simulink model "pemfc_lumpekf2_prerun_2"  (R2021b)
settings: Solver=ode3  StartTime=0.0  StopTime=10  FixedStep=0.001  MaxStep=dt  RelTol=1e-6
values from neighbouring files (symbols this model uses):
  Optparameter = [kp,kd,ki,b,m1,m2,delta]    [OptGain.m]
  P0 = diag([10,10,10000,10000,10000])    [input_sine.m]    (also in input_step.m)
  x0 = [0.21;0.21;1;1;1]    [OptGain.m]    (also in input_sine.m = [xch_O2c;xch_O2c;J_ss;J_ss;J_ss]; input_step.m = [xch_O2c;xch_O2c;J_ss;J_ss;J_ss])
  xhat0 = [0;0;0;0;0]    [input_sine.m]    (also in input_step.m)
settings Model: Creator=kvijayar  LastModifiedBy=AlirezaBeigi
settings SolverCC: AlgebraicLoopSolver=TrustRegion
settings DataIOCC: InitialState=AA
settings DebuggingCC: SFMachineParentedDataDiag=warning

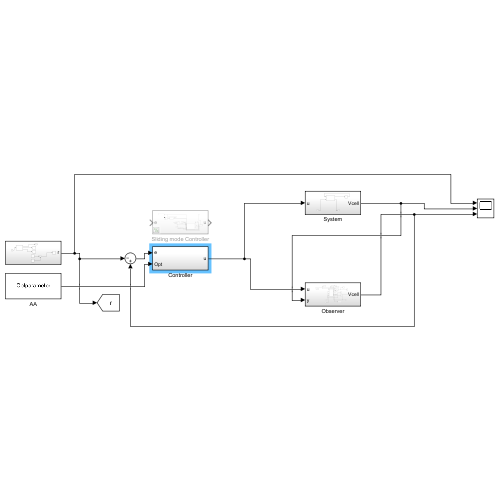
[thumbnail: Simulink's stored preview of the top-level diagram]
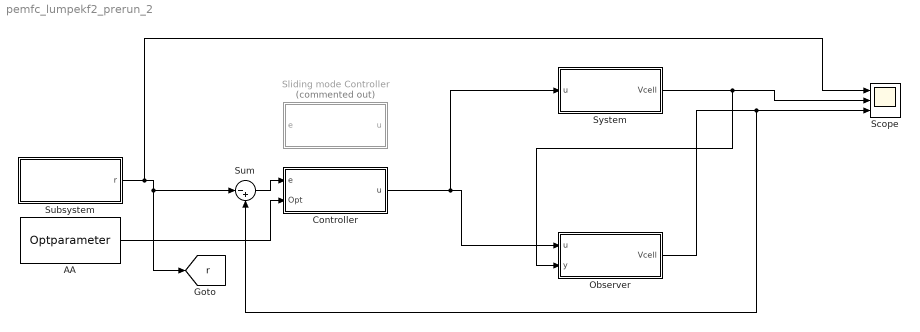
== system pemfc_lumpekf2_prerun_2 ==
  AA : Constant  Value=Optparameter  SampleTime=-1
  Controller : Subsystem  Tag=Controller  Description=Controller
  Observer : Subsystem
  Scope : Scope  NumInputPorts=3
  Sliding mode Controller : Subsystem  Commented=on
  Subsystem : Subsystem
  Sum : Sum  Inputs=|-+
  System : Subsystem
  tag scope: r=global
  wires:
  System/1(Vcell) -> Scope/2, Observer/2(y)
  Observer/1(Vcell) -> Scope/3, Sum/2
  Subsystem/1(r) -> Scope/1, Sum/1, [r]
  Sum/1 -> Controller/1(e)
  Controller/1(u) -> System/1(u), Observer/1(u)
  AA/1 -> Controller/2(Opt)

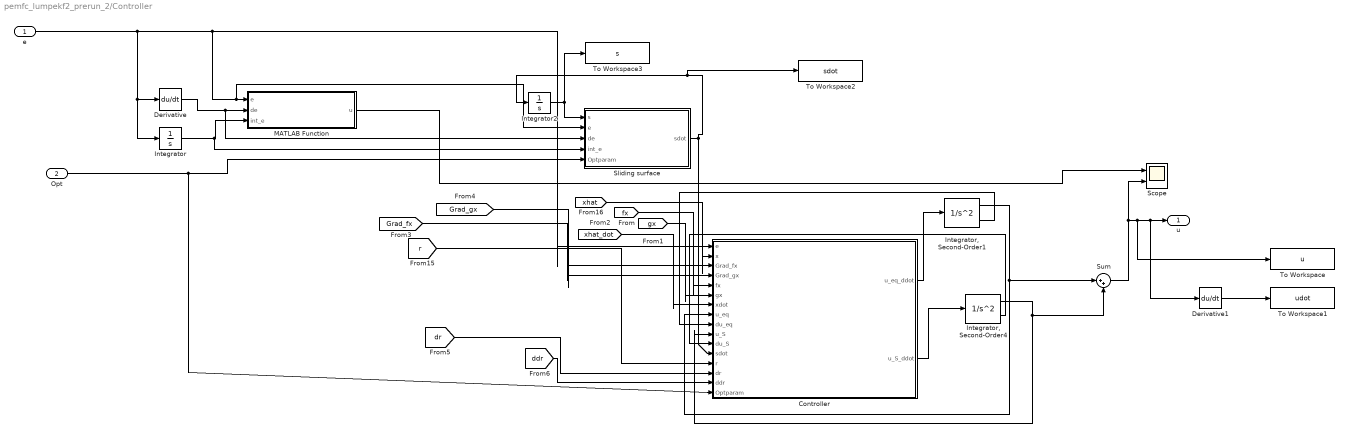
== system pemfc_lumpekf2_prerun_2/Controller ==
  e : Inport
  Opt : Inport  Port=2
  Controller : MATLAB Function  TreatAsAtomicUnit=on
  Derivative : Derivative  CoefficientInTFapproximation=0
  Derivative1 : Derivative  CoefficientInTFapproximation=0
  Integrator : Integrator
  "Integrator, Second-Order1" : SecondOrderIntegrator  ICX=8
  "Integrator, Second-Order4" : SecondOrderIntegrator
  Integrator2 : Integrator
  MATLAB Function : MATLAB Function  TreatAsAtomicUnit=on
  Scope : Scope  NumInputPorts=2
  Sliding surface : MATLAB Function  TreatAsAtomicUnit=on
  Sum : Sum  Inputs=|++
  To Workspace : ToWorkspace  VariableName=u  SaveFormat=Timeseries  SampleTime=-1
  To Workspace1 : ToWorkspace  VariableName=udot  SaveFormat=Timeseries  SampleTime=-1
  To Workspace2 : ToWorkspace  VariableName=sdot  SaveFormat=Timeseries  SampleTime=-1
  To Workspace3 : ToWorkspace  VariableName=s  SaveFormat=Timeseries  SampleTime=-1
  u : Outport
  wires:
  e/1 -> Controller/1(e), Sliding surface/2(e), MATLAB Function/1(e), Integrator/1, Derivative/1
  Derivative/1 -> Sliding surface/3(de), MATLAB Function/2(de)
  Integrator/1 -> Sliding surface/4(int_e), MATLAB Function/3(int_e)
  Integrator2/1 -> To Workspace3/1, Sliding surface/1(s)
  [r] -> Controller/13(r)
  [xhat] -> Controller/2(x)
  Controller/1(u_eq_ddot) -> "Integrator, Second-Order1"/1
  Controller/2(u_S_ddot) -> "Integrator, Second-Order4"/1
  "Integrator, Second-Order4"/1 -> Sum/2, Controller/10(u_S)
  "Integrator, Second-Order4"/2 -> Controller/11(du_S)
  [fx] -> Controller/5(fx)
  [gx] -> Controller/6(gx)
  [xhat_dot] -> Controller/7(xdot)
  [Grad_gx] -> Controller/4(Grad_gx)
  [Grad_fx] -> Controller/3(Grad_fx)
  "Integrator, Second-Order1"/1 -> Sum/1, Controller/8(u_eq)
  "Integrator, Second-Order1"/2 -> Controller/9(du_eq)
  [ddr] -> Controller/15(ddr)
  [dr] -> Controller/14(dr)
  MATLAB Function/1(u) -> Scope/1
  Sum/1 -> To Workspace/1, Derivative1/1, u/1, Scope/2
  Derivative1/1 -> To Workspace1/1
  Sliding surface/1(sdot) -> To Workspace2/1, Integrator2/1, Controller/12(sdot)
  Opt/1 -> Controller/16(Optparam), Sliding surface/5(Optparam)

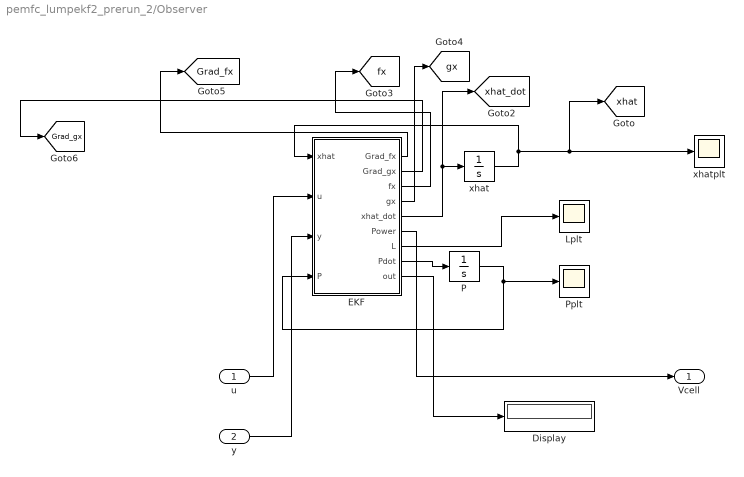
== system pemfc_lumpekf2_prerun_2/Observer ==
  u : Inport
  y : Inport  Port=2
  Display : Display
  EKF : MATLAB Function  TreatAsAtomicUnit=on
  Lplt : Scope
  P : Integrator  InitialCondition=P0
  Pplt : Scope
  xhat : Integrator  InitialCondition=xhat0
  xhatplt : Scope
  Vcell : Outport
  tag scope: Grad_fx=global, Grad_gx=global, fx=global, gx=global, xhat=global, xhat_dot=global
  wires:
  EKF/8(Pdot) -> P/1
  P/1 -> Pplt/1, EKF/4(P)
  xhat/1 -> [xhat], xhatplt/1, EKF/1(xhat)
  EKF/5(xhat_dot) -> [xhat_dot], xhat/1
  EKF/7(L) -> Lplt/1
  EKF/6(Power) -> Vcell/1
  u/1 -> EKF/2(u)
  y/1 -> EKF/3(y)
  EKF/3(fx) -> [fx]
  EKF/4(gx) -> [gx]
  EKF/1(Grad_fx) -> [Grad_fx]
  EKF/2(Grad_gx) -> [Grad_gx]
  EKF/9(out) -> Display/1

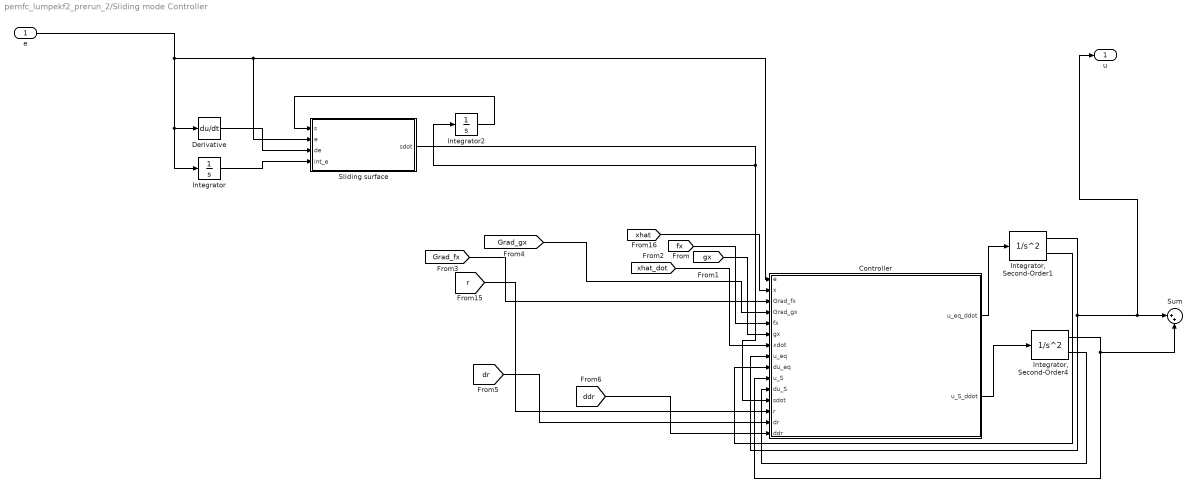
== system pemfc_lumpekf2_prerun_2/Sliding mode Controller ==
  e : Inport
  Controller : MATLAB Function  TreatAsAtomicUnit=on
  Derivative : Derivative  CoefficientInTFapproximation=0
  Integrator : Integrator
  "Integrator, Second-Order1" : SecondOrderIntegrator  AbsoluteToleranceX=0.01
  "Integrator, Second-Order4" : SecondOrderIntegrator
  Integrator2 : Integrator
  Sliding surface : MATLAB Function  TreatAsAtomicUnit=on
  Sum : Sum  Inputs=|++
  u : Outport
  wires:
  Derivative/1 -> Sliding surface/3(de)
  "Integrator, Second-Order1"/1 -> u/1, Sum/1, Controller/8(u_eq)
  [ddr] -> Controller/15(ddr)
  "Integrator, Second-Order1"/2 -> Controller/9(du_eq)
  [Grad_fx] -> Controller/3(Grad_fx)
  [dr] -> Controller/14(dr)
  [gx] -> Controller/6(gx)
  Controller/1(u_eq_ddot) -> "Integrator, Second-Order1"/1
  Controller/2(u_S_ddot) -> "Integrator, Second-Order4"/1
  [fx] -> Controller/5(fx)
  [Grad_gx] -> Controller/4(Grad_gx)
  [xhat] -> Controller/2(x)
  "Integrator, Second-Order4"/1 -> Sum/2, Controller/10(u_S)
  "Integrator, Second-Order4"/2 -> Controller/11(du_S)
  Integrator2/1 -> Sliding surface/1(s)
  [xhat_dot] -> Controller/7(xdot)
  Integrator/1 -> Sliding surface/4(int_e)
  [r] -> Controller/13(r)
  Sliding surface/1(sdot) -> Controller/12(sdot), Integrator2/1
  e/1 -> Controller/1(e), Sliding surface/2(e), Integrator/1, Derivative/1

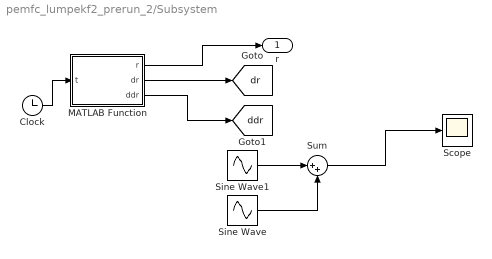
== system pemfc_lumpekf2_prerun_2/Subsystem ==
  Clock : Clock
  MATLAB Function : MATLAB Function  TreatAsAtomicUnit=on
  Scope : Scope
  Sine Wave : Sin  Amplitude=3  Bias=4  Frequency=4  SampleTime=0
  Sine Wave1 : Sin  Amplitude=5  Bias=2  Frequency=2  SampleTime=0
  Sum : Sum  Inputs=|++
  r : Outport
  tag scope: ddr=global, dr=global
  wires:
  Sine Wave1/1 -> Sum/1
  Sine Wave/1 -> Sum/2
  Sum/1 -> Scope/1
  Clock/1 -> MATLAB Function/1(t)
  MATLAB Function/1(r) -> r/1
  MATLAB Function/2(dr) -> [dr]
  MATLAB Function/3(ddr) -> [ddr]

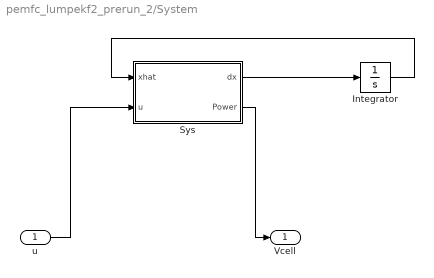
== system pemfc_lumpekf2_prerun_2/System ==
  u : Inport
  Integrator : Integrator  InitialCondition=x0
  Sys : MATLAB Function  TreatAsAtomicUnit=on
  Vcell : Outport
  wires:
  u/1 -> Sys/2(u)
  Sys/1(dx) -> Integrator/1
  Integrator/1 -> Sys/1(xhat)
  Sys/2(Power) -> Vcell/1

== matlab function pemfc_lumpekf2_prerun_2/Controller/Controller ==
  data: e input; x input; Grad_fx input; Grad_gx input; fx input; gx input; xdot input; u_eq input; du_eq input; u_S input; du_S input; u_eq_ddot output; sdot input; r input; dr input; ddr input; u_S_ddot output; Optparam input
function [u_eq_ddot,u_S_ddot] = controller(e,x,Grad_fx,Grad_gx,fx,gx,xdot,u_eq,du_eq,u_S,du_S,sdot,r,dr,ddr,Optparam)
u_eq_ddot = 4.;
u_S_ddot = 4.;
%% Setting up Control parameter 

kp = double(Optparam(1));kd =  double(Optparam(2));ki = double(Optparam(3));b =  double(Optparam(4));m1 =  double(Optparam(5));m2 =  double(Optparam(6));delta =  double(Optparam(7));

q = 5;
p = 3;

alpha = 0.9;

u = u_eq + u_S;

%% Setting up System parameter 
param.xO2normal = 0.22;
param.BV_Vact0 = 0.0178;
param.J_lim = 30000;
param.BV_J0 = 0.006;
param.Bconc = 0.05;
param.E0_cell = 1.2271;
param.w = 0.05;
param.kE=1.7708e-05;
param.Tfc = 273+33;
	param.r1 = 0.006;
	param.r2 = 4.0000e-05;
	param.rt = 5.0000e-05;
    xch_O2c=0.21;
    param.lc = 1;
    xch_H2a=0.99;
    Pa = 1.5;	%In atm
	Pc = 1; %atm.
J_in = u;
L_zFD=param.xO2normal/param.J_lim;
phi_avg = Pc*xch_O2c;
phiH2_in = Pa*xch_H2a;
phi_eff = 0.1512*phi_avg + 4/pi*x(1) - 4/(3*pi)*x(2) ...
        - (0.1894*J_in + 8/pi^2*x(3))*L_zFD;
J_act = x(5);

temp = [(4/pi)^2,-(1/3)*(4/pi)^2,(4/pi)*(8/pi^2),0,(4/pi)*(-0.1894);
    (1/3)*(4/pi)^2,-(1/9)*(4/pi)^2,(4/pi)*(8/pi^2),0,(4/(3.*pi))*(-0.1894);
    -L_zFD*(4/(pi))*(8/pi^2),-L_zFD*(4/(3.*pi))*(8/pi^2),-L_zFD*(8/(pi))*(8/pi^2),0,-L_zFD*(-0.1894)*(8/pi^2);
    0,0,0,0,0;
     -L_zFD*(-0.1894)*(4/(pi)),-L_zFD*(-0.1894)*(4/(3*pi)),-L_zFD*(-0.1894)*(8/(pi)^2),0,-L_zFD*(-0.1894)*(8/(pi)^2)+2*param.BV_Vact0*J_act/sqrt( 4*param.BV_J0^2 + J_act^2 )];
Gradhxx = u*(-param.Bconc/phi_eff)*temp;
Gradhx = u*[(param.Bconc*(4/pi)/phi_eff);
    (-param.Bconc*(4/(3*pi))/phi_eff);
    (-param.Bconc*(8/pi^2)*L_zFD/phi_eff);
    0;
    -param.Bconc*L_zFD*(0.1894)/(phi_eff) - 2*param.BV_Vact0/sqrt( 4*param.BV_J0^2 + J_act^2 )];
Gradhux = [(param.Bconc*(4/pi)/phi_eff);
    (-param.Bconc*(4/(3*pi))/phi_eff);
    (-param.Bconc*(8/pi^2)*L_zFD/phi_eff);
    0;
    -param.Bconc*L_zFD*(0.1894)/(phi_eff) - 2*param.BV_Vact0/sqrt( 4*param.BV_J0^2 + J_act^2 )];

Area = param.lc*param.w;
I = J_in*Area;
    E0T = param.E0_cell - param.kE*(param.Tfc-298);
    Vact = 2*param.BV_Vact0*asinh(J_act/(2*param.BV_J0));
    if phi_eff<0
        Econc = 0;
    else
        Econc = 2*param.Bconc*log(phiH2_in) + param.Bconc*log(real(phi_eff));
    end
    
    Ecellc =  E0T +  Econc;
    Vohm = (param.r1*I+ param.r2*I^2 - param.rt*(param.Tfc-298)*I); 
    

Gradhu = (Ecellc - Vohm - Vact)+ Area*(param.r1*2.*u+ 3.*param.r2*u^2 - 2.*param.rt*(param.Tfc-298)*u);  
Gradhuu =  Area*(param.r1*2.*u+ 3.*param.r2*u^2 - 2.*param.rt*(param.Tfc-298)*u) + Area*(param.r1*2+ 6*param.r2*u - 2.*param.rt*(param.Tfc-298)); 
Gradhxu = [(param.Bconc*(4/pi)/phi_eff);
    (-param.Bconc*(4/(3*pi))/phi_eff);
    (-param.Bconc*(8/pi^2)*L_zFD/phi_eff);
    0;
    -param.Bconc*L_zFD*(0.1894)/(phi_eff) - 2*param.BV_Vact0/sqrt( 4*param.BV_J0^2 + J_act^2 )];
% t1 = (fx + gx*u_eq)'*Gradhxx*(fx + gx*u_eq)
% t2 = Gradhxx
% t3 = (fx + gx*u_eq)
% t4 = kd*(2*du_eq*Gradhux'*(fx + gx*u_eq) + Gradhx'*(Grad_fx'*xdot + Grad_gx'*xdot*u_eq)+ Gradhuu*du_eq^2-ddr-b*sdot )
% t5 = Gradhx'*(Grad_fx'*xdot + Grad_gx'*xdot*u_eq)
% t6 = Gradhuu*du_eq^2-ddr-b*sdot
% t7 = kp*(Gradhx'*(fx + gx*u_eq)+Gradhu*du_eq - dr)
% t8 = +ki*(sign(e)*abs(e)^(q/p))

u_eq_ddot = -(Gradhu/((Gradhu)^2 + 0.0001))*(kp*(Gradhx'*(fx + gx*u_eq)+Gradhu*du_eq - dr)+ki*(sign(e)*abs(e)^(q/p))+kd*( ...
   2*du_eq*Gradhux'*(fx + gx*u_eq) + Gradhx'*(Grad_fx'*xdot + Grad_gx'*xdot*u_eq)+ Gradhuu*du_eq^2-ddr-b*sdot ));


%%(fx + gx*u_eq)'*Gradhxx*(fx + gx*u_eq)+
%u_eq_ddot = -(Gradhu/((Gradhu)^2 + 0.0001))*(kp*(Gradhx'*(fx + gx*u_eq)+Gradhu*du_eq - dr)+ki*(sign(e)*abs(e)^(q/p))+kd*((fx + gx*u_eq)'*Gradhxx*(fx + gx*u_eq)+ ...
%    2*du_eq*Gradhux'*(fx + gx*u_eq) + Gradhx'*(Grad_fx'*xdot + Grad_gx'*xdot*u_eq)+ Gradhuu*du_eq^2-ddr-b*sdot ))
%u_eq_ddot = 0;
u_S_ddot =  -(Gradhu/((Gradhu)^2 + 0.0001))*(kp*(Gradhx'*(gx*u_S)+Gradhu*du_S)+kd*((gx*u_S)'*Gradhxx*(gx*u_S))+(gx*u_S)'*Gradhxu*du_S ...
    +Gradhuu*du_S^2+Gradhx'*(Grad_gx'*xdot)*u_S+m1*abs(sdot)*sign(sdot)+m2*sign(sdot)*abs(sdot)^alpha+delta*sign(sdot));

== matlab function pemfc_lumpekf2_prerun_2/Sliding mode Controller/Sliding surface ==
  data: s input; sdot output; e input; de input; int_e input
function sdot = SurfaceCal(s,e,de,int_e)
kp = 40;
kd = 0.002;
ki = 0.1;
b = 5.;
sdot = -b*s + kp*e + ki*int_e + kd*de;

== matlab function pemfc_lumpekf2_prerun_2/Subsystem/MATLAB Function ==
  data: t input; r output; dr output; ddr output
function [r, dr, ddr] = desired(t)
r = + 5.*cos(t)+ 3.*sin(3*t);
dr = -5.*sin(t) + 9.*cos(3.*t);
ddr = 5.*cos(t) - 27.*sin(3.*t);

== matlab function pemfc_lumpekf2_prerun_2/Observer/EKF ==
  data: Grad_fx output; Grad_gx output; fx output; gx output; xhat_dot output; Power output; xhat input; u input; y input; L output; P input; Pdot output; param parameter; out output
function [Grad_fx,Grad_gx,fx,gx,xhat_dot,Power, L,Pdot,out] = EKF(xhat,u,y,P, param)

    x = xhat;
    J_in = u;
    slm = 1/24.4/60;
    Ndot_a = 1.03*slm;
    Ndot_c = 1.03*slm;
    xch_O2c=0.21;
    xch_H2a=0.99;
    Pa = 1.5;	%In atm
	Pc = 1; %atm.
    phiH2_in = Pa*xch_H2a;
    phiO2_in = Pc*xch_O2c;
%%Common
    %x=[ϕ_0,ϕ_1,J_0,J_1,J_act ]^T --> change J to current?; u(1),u(2),ϕ_0,ϕ_1 are partial presure
    %u = [ϕ_(H2,A)^in, ϕ_(o2,C)^in, J]';
    %τ_m=1/(Dλ_m^2 )=τ_0/(2m+1)^2 
    tau0_1 = 1/param.tau_flux_O2;
    tau1_1 = 9*tau0_1; %tau0/(2*1+1)^2
    J_act = x(5);
    Area = param.lc*param.w;
    I = J_in*Area;
    %tauact = √(4J_0^2+(J_act )^2 )/(2V_(act,0) C_DL/Area)
    tauact_1 = Area*sqrt( 4*param.BV_J0^2 + J_act^2 )/( 2*param.BV_Vact0*param.Cdbl );
    tauactH2_1 = Area*sqrt( 4*param.BV_JH20^2 + J_act^2 )/( 2*param.BV_VactH20*param.Cdbl );
    
    %[4J_0^2+2J_act^2-J J_act ]/(4J_0^2+J_act^2 )
    tauact_ekf= tauact_1*( 4*param.BV_J0^2 + 2*J_act^2 - J_in*J_act)/( 4*param.BV_J0^2 + J_act^2 );
    tauactH2_ekf=tauactH2_1*( 4*param.BV_JH20^2 + 2*J_act^2 - J_in*J_act)/( 4*param.BV_JH20^2 + J_act^2 );
    %%EKF
    %f=param.ekf.f;
    Tch=( 0.1512*J_in + 4/pi*x(3) - 4/(3*pi)*x(4) )*Area/(4*param.Ndot_c*param.F); %Γ_ch≔J̅/nF --> (J̅A)⁄(4Ṅ_C F)
    phiO2_out = param.Pc - (param.Pc-phiO2_in)/(1-Tch);
    if param.ekf.f >= 0
        f=param.ekf.f;
    else
        if (phiO2_out>0)
            f=0.5;
        else
            %Find at what what point in channel phiO2_out=0
            %(Tch) = (phiO2_in/param.Pc);
            %phi_avg = f*phiO2_in+(1-f)*phiO2_out; --> f % of inlet in blend
            fend=phiO2_in/param.Pc/Tch;
            f=fend/2;
        end
    end
    f_ = 1;
    L_zFD=param.xO2normal/param.J_lim;
    
    h_H2=(1-f*J_in*Area/(2*Ndot_a*param.F))/(1-J_in*Area/(2*Ndot_a*param.F));
    h_H2J=(1-f)*(param.Pc-phiH2_in)/(1-J_in*Area/(2*Ndot_a*param.F))^2*Area/(2*Ndot_a*param.F);
    h_H2N=h_H2J*J_in/Ndot_a;
    
    %0.1512J_act+4/π J_0-4/3π J_1
    Jbar=0.1512*x(5)+4/pi*x(3)-4/(3*pi)*x(4);
    %h_O2=(1-f (J ̅A)⁄(4N ̇_C param.F))/(1-(J ̅A)⁄(4N ̇_C param.F)),
    h_O2=(1-f*Jbar*Area/(4*Ndot_c*param.F))/(1-Jbar*Area/(4*Ndot_c*param.F));
    %h_O2J=(1-f)(P_A-ϕ_(O2,C)^in )/(1-(J ̅A)⁄(4N ̇_C param.F))^2   Area/(4N ̇_C param.F),
    h_O2J=(1-f)*(param.Pa-phiO2_in)/(1-Jbar*Area/(4*Ndot_c*param.F))^2*Area/(4*Ndot_c*param.F);
    %h_O2N=(h_O2J J ̅)/N ̇_C
    h_O2N=h_O2J*Jbar/Ndot_c;

    phiO2_1.MO2avg=0.1512*h_O2J *[0 0 4/pi -4/(3*pi) 0.1512];
    phiO2_1.MO2avgU = [0 h_O2 0 0 h_O2N];

    f_ = 1;
    MO2avg=f_*phiO2_1.MO2avg;
    MO2avgU=f_*phiO2_1.MO2avgU;
    phi_avg = f*phiO2_in;
        
    MO2eff= MO2avg+[4/pi -4/(3*pi) -8/pi^2*L_zFD 0 -0.1894*L_zFD];
    MO2effU=0.1512*MO2avgU;

    %ϕ_(O2,eff)=[0.1512×ϕ_(O2-ch)-4/π ϕ_0+4/3π ϕ_1 ]-[0.1894J-8/π^2  J_0 ]×L/zFD
    %Assume phi_nom - Jlim*L/(zFD) = 0 OR L/(zFD) = phi_nom/J_lim
    phi_eff = 0.1512*phi_avg + 4/pi*x(1) - 4/(3*pi)*x(2) ...
        - (0.1894*J_in + 8/pi^2*x(3))*L_zFD;
    Vohm = (param.r1*I+ param.r2*I^2 - param.rt*(param.Tfc-298)*I);  

%% EKF A,B,C,D
    %Non-zero
    phieff_1.A=...
		 -diag([tau0_1,tau1_1,tau0_1,tau1_1,tauact_ekf])...
            +[zeros(5,4),[0;0;tau0_1;tau1_1;0]]...
            +[tau0_1*MO2avg;tau1_1*MO2avg;zeros(3,5)];
    phieff_1.B=...
		[ tau0_1*MO2avgU;
            tau1_1*MO2avgU;
            0   0   0   0   0;
            0   0   0   0   0;
            0   0   tauact_1    0   0];
    phieff_1.C=param.Bconc*phi_eff*MO2eff...
            -2*param.BV_Vact0/sqrt( 4*param.BV_J0^2 + J_act^2 )*[0 0 0 0 1];
    phieff_1.D=2*param.Bconc/(phiH2_in)*[h_H2 0 h_H2J -h_H2N 0]...
            + param.Bconc/(phi_eff)*MO2effU...
            + [0 0 -(param.r1+ param.r2*I - param.rt*(param.Tfc-298))*Area 0 0];
    phieff_1.Vact=2*param.BV_Vact0*asinh(J_act*Area/(2*param.BV_I0));
    phieff_1.Ecellc=0;
    %phieff_1.Ecellc=param.E0_cell;% - param.kE*(param.Tfc-298) ...
    %       + 2*param.Bconc*log(phiH2_in) + param.Bconc*log(phi_eff) ;
    
    %Zero
    phieff_0.A=-diag([tau0_1,tau1_1,tau0_1,tau1_1,tauactH2_1])...
            +[zeros(5,4),[0;0;tau0_1;tau1_1;0]];
    phieff_0.B=...
		[ tau0_1*MO2avgU;
            tau1_1*MO2avgU;
            0   0   0   0   0;
            0   0   0   0   0;
            0   0   tauactH2_ekf    0   0];
    phieff_0.C=-2*param.BV_VactH20/sqrt( 4*param.BV_JH20^2 + J_act^2 )*[0 0 0 0 1];
    phieff_0.D=[0 0 -(param.r1+ param.r2*I - param.rt*(param.Tfc-298))*Area 0 0];
    phieff_0.Vact=...
		 2*param.BV_VactH20*asinh(J_act/(2*param.BV_JH20));
    phieff_0.Ecellc=0;
    phieff.f = 1;

%% Cell output
    %%System x dot
    E0T = param.E0_cell - param.kE*(param.Tfc-298);
    %phi_eff > 0
    phieff_1.dx = [
        tau0_1*( phi_avg - x(1) );
        tau1_1*( phi_avg - x(2) );
        tau0_1*( x(5) - x(3) );
        tau1_1*( x(5) - x(4) );
        tauact_1*( J_in - x(5) )
    ];
    phieff_1.Vact = 2*param.BV_Vact0*asinh(J_act/(2*param.BV_J0));
    if phi_eff<0
        phieff_1.Econc = 0;
    else
        phieff_1.Econc = 2*param.Bconc*log(phiH2_in) + param.Bconc*log(real(phi_eff));
    end

    phieff_1.Ecellc =  E0T +  phieff_1.Econc;
    fx = [
        tau0_1*( phi_avg - x(1) );
        tau1_1*( phi_avg - x(2) );
        tau0_1*( x(5) - x(3) );
        tau1_1*( x(5) - x(4) );
        tauact_1*(  - x(5) );
    ];

    gx = [
        0;
        0;
        0;
        0;
        tauact_1;
    ];
 
    
%% Final
    %EKF
    f_=phieff.f;
    A = f_*phieff_1.A ;
    B = f_*phieff_1.B ;
    C = f_*phieff_1.C ;
    D = f_*phieff_1.D ;
    Rsys=0.1^2;Qsys=diag([0.1^2 0.021^2 0.1^2/Area^2]);
Qsys=diag([diag(Qsys);0.01*param.Ndot_a;0.01*param.Ndot_c]);

    Qb = B*Qsys*B';
    Rb = Rsys+D*Qsys*D';

    Pdot = A*P+P*A'-P*C'*(Rb)^-1*C*P+Qb;

    L = P*C'*(Rb)^-1;
    
    %Cell output
    Grad_fx = phieff_1.A;
    Grad_gx = phieff_1.B;
    Econc = f_*phieff_1.Econc ;
    Ecellc = f_*phieff_1.Ecellc ;
    Vact = f_*phieff_1.Vact ;
    dx = f_*phieff_1.dx ;


    Power = u*(Ecellc - Vohm - Vact);
    xhat_dot = dx + L*(y-Power);
    out = [phi_eff,phi_avg,phiO2_out,Ecellc,Vohm,Vact,E0T,Econc];
    %out.phi_eff = phi_eff;

== matlab function pemfc_lumpekf2_prerun_2/Controller/MATLAB Function ==
  data: e input; u output; de input; int_e input
function u = PIDcontroller(e, de, int_e)
kp = 100000;
kd = 100;
ki = 10;

u = kp*e+kd*de+ki*int_e;

== matlab function pemfc_lumpekf2_prerun_2/System/Sys ==
  data: dx output; Power output; xhat input; u input; param parameter
function [dx,Power] = Sys(xhat,u, param)
    
    x = xhat;
    J_in=u;
    slm = 1/24.4/60;
    Ndot_a = 1.03*slm;
    Ndot_c = 1.03*slm;
    xch_O2c=0.21;
    xch_H2a=0.99;
    Pa = 1.5;	%In atm
	Pc = 1; %atm.
    phiH2_in = Pa*xch_H2a;
    phiO2_in = Pc*xch_O2c;

%%Common
    %x=[ϕ_0,ϕ_1,J_0,J_1,J_act ]^T --> change J to current?; u(1),u(2),ϕ_0,ϕ_1 are partial presure
    %u = [ϕ_(H2,A)^in, ϕ_(o2,C)^in, J]';
    %τ_m=1/(Dλ_m^2 )=τ_0/(2m+1)^2 
    tau0_1 = 1/param.tau_flux_O2;
    tau1_1 = 9*tau0_1; %tau0/(2*1+1)^2
    J_act = x(5);
    Area = param.lc*param.w;
    I = J_in*Area;
    %tauact = √(4J_0^2+(J_act )^2 )/(2V_(act,0) C_DL/Area)
    tauact_1 = Area*sqrt( 4*param.BV_J0^2 + J_act^2 )/( 2*param.BV_Vact0*param.Cdbl );
    tauactH2_1 = Area*sqrt( 4*param.BV_JH20^2 + J_act^2 )/( 2*param.BV_VactH20*param.Cdbl );
    
    %[4J_0^2+2J_act^2-J J_act ]/(4J_0^2+J_act^2 )
    tauact_ekf= tauact_1*( 4*param.BV_J0^2 + 2*J_act^2 - J_in*J_act)/( 4*param.BV_J0^2 + J_act^2 );
    tauactH2_ekf=tauactH2_1*( 4*param.BV_JH20^2 + 2*J_act^2 - J_in*J_act)/( 4*param.BV_JH20^2 + J_act^2 );
    %%EKF
    %f=param.ekf.f;
    Tch=( 0.1512*J_in + 4/pi*x(3) - 4/(3*pi)*x(4) )*Area/(4*param.Ndot_c*param.F); %Γ_ch≔J̅/nF --> (J̅A)⁄(4Ṅ_C F)
    phiO2_out = param.Pc - (param.Pc-phiO2_in)/(1-Tch);
    if param.ekf.f >= 0
        f=param.ekf.f;
    else
        if (phiO2_out>0)
            f=0.5;
        else
            %Find at what what point in channel phiO2_out=0
            %(Tch) = (phiO2_in/param.Pc);
            %phi_avg = f*phiO2_in+(1-f)*phiO2_out; --> f % of inlet in blend
            fend=phiO2_in/param.Pc/Tch;
            f=fend/2;
        end
    end
    f_ = 1;
    L_zFD=param.xO2normal/param.J_lim;
    
    h_H2=(1-f*J_in*Area/(2*Ndot_a*param.F))/(1-J_in*Area/(2*Ndot_a*param.F));
    h_H2J=(1-f)*(param.Pc-phiH2_in)/(1-J_in*Area/(2*Ndot_a*param.F))^2*Area/(2*Ndot_a*param.F);
    h_H2N=h_H2J*J_in/Ndot_a;
    
    %0.1512J_act+4/π J_0-4/3π J_1
    Jbar=0.1512*x(5)+4/pi*x(3)-4/(3*pi)*x(4);
    %h_O2=(1-f (J ̅A)⁄(4N ̇_C param.F))/(1-(J ̅A)⁄(4N ̇_C param.F)),
    h_O2=(1-f*Jbar*Area/(4*Ndot_c*param.F))/(1-Jbar*Area/(4*Ndot_c*param.F));
    %h_O2J=(1-f)(P_A-ϕ_(O2,C)^in )/(1-(J ̅A)⁄(4N ̇_C param.F))^2   Area/(4N ̇_C param.F),
    h_O2J=(1-f)*(param.Pa-phiO2_in)/(1-Jbar*Area/(4*Ndot_c*param.F))^2*Area/(4*Ndot_c*param.F);
    %h_O2N=(h_O2J J ̅)/N ̇_C
    h_O2N=h_O2J*Jbar/Ndot_c;

    phiO2_1.MO2avg=0.1512*h_O2J *[0 0 4/pi -4/(3*pi) 0.1512];
    phiO2_1.MO2avgU = [0 h_O2 0 0 h_O2N];
    phiO2_0.MO2avg=zeros(1,5);
    phiO2_0.MO2avgU = [0 f 0 0 0];

    f_ = 1;
    MO2avg=f_*phiO2_1.MO2avg;
    MO2avgU=f_*phiO2_1.MO2avgU;

    phi_avg = f*phiO2_in;
        
    MO2eff= MO2avg+[4/pi -4/(3*pi) -8/pi^2*L_zFD 0 -0.1894*L_zFD];
    MO2effU=0.1512*MO2avgU;

    %ϕ_(O2,eff)=[0.1512×ϕ_(O2-ch)-4/π ϕ_0+4/3π ϕ_1 ]-[0.1894J-8/π^2  J_0 ]×L/zFD
    %Assume phi_nom - Jlim*L/(zFD) = 0 OR L/(zFD) = phi_nom/J_lim
    phi_eff = 0.1512*phi_avg + 4/pi*x(1) - 4/(3*pi)*x(2) ...
        - (0.1894*J_in + 8/pi^2*x(3))*L_zFD;
    Vohm = (param.r1*I+ param.r2*I^2 - param.rt*(param.Tfc-298)*I);  

%% EKF A,B,C,D
    %Non-zero
    phieff_1.A=...
		 -diag([tau0_1,tau1_1,tau0_1,tau1_1,tauact_ekf])...
            +[zeros(5,4),[0;0;tau0_1;tau1_1;0]]...
            +[tau0_1*MO2avg;tau1_1*MO2avg;zeros(3,5)];
    phieff_1.B=...
		[ tau0_1*MO2avgU;
            tau1_1*MO2avgU;
            0   0   0   0   0;
            0   0   0   0   0;
            0   0   tauact_1    0   0];
    phieff_1.C=param.Bconc*phi_eff*MO2eff...
            -2*param.BV_Vact0/sqrt( 4*param.BV_J0^2 + J_act^2 )*[0 0 0 0 1];
    phieff_1.D=2*param.Bconc/(phiH2_in)*[h_H2 0 h_H2J -h_H2N 0]...
            + param.Bconc/(phi_eff)*MO2effU...
            + [0 0 -(param.r1+ param.r2*I - param.rt*(param.Tfc-298))*Area 0 0];
    phieff_1.Vact=2*param.BV_Vact0*asinh(J_act*Area/(2*param.BV_I0));
    phieff_1.Ecellc=0;
    %phieff_1.Ecellc=param.E0_cell;% - param.kE*(param.Tfc-298) ...
    %       + 2*param.Bconc*log(phiH2_in) + param.Bconc*log(phi_eff) ;
    
    %Zero
    phieff_0.A=-diag([tau0_1,tau1_1,tau0_1,tau1_1,tauactH2_1])...
            +[zeros(5,4),[0;0;tau0_1;tau1_1;0]];
    phieff_0.B=...
		[ tau0_1*MO2avgU;
            tau1_1*MO2avgU;
            0   0   0   0   0;
            0   0   0   0   0;
            0   0   tauactH2_ekf    0   0];
    phieff_0.C=-2*param.BV_VactH20/sqrt( 4*param.BV_JH20^2 + J_act^2 )*[0 0 0 0 1];
    phieff_0.D=[0 0 -(param.r1+ param.r2*I - param.rt*(param.Tfc-298))*Area 0 0];
    phieff_0.Vact=...
		 2*param.BV_VactH20*asinh(J_act/(2*param.BV_JH20));
    phieff_0.Ecellc=0;
    if phi_eff > param.sim.phieff_eps
        phieff.f = 1;
    else
        if phi_eff < 0
            phi_eff = 0;
        end
        phieff.f = phi_eff/param.sim.phieff_eps;
    end
    phieff.f = 1;
    %y = 0.5*param.Bconc*log(phi_eff) - 2*param.BV_Vact0*asinh(J_act*Area/(2*param.BV_I0));
    %Vcell = Ecellc - Vohm - Vact;
%% Cell output
    %%System x dot
    E0T = param.E0_cell - param.kE*(param.Tfc-298);
    %phi_eff > 0
    phieff_1.dx = [
        tau0_1*( phi_avg - x(1) );
        tau1_1*( phi_avg - x(2) );
        tau0_1*( x(5) - x(3) );
        tau1_1*( x(5) - x(4) );
        tauact_1*( J_in - x(5) )
    ];

    phieff_1.Vact = 2*param.BV_Vact0*asinh(J_act/(2*param.BV_J0));
    phieff_1.Econc = 2*param.Bconc*log(phiH2_in) + param.Bconc*log(phi_eff);
    phieff_1.Ecellc =  E0T +  phieff_1.Econc;

    
%% Final
    %EKF
    f_=phieff.f;


    %Cell output

    Ecellc = f_*phieff_1.Ecellc ;
    Vact = f_*phieff_1.Vact ;
    dx = f_*phieff_1.dx ;

    Power = u*(Ecellc - Vohm - Vact);


    %out.phi_eff = phi_eff;

== matlab function pemfc_lumpekf2_prerun_2/Controller/Sliding surface ==
  data: s input; sdot output; e input; de input; int_e input; Optparam input
function sdot = SurfaceCal(s, e, de, int_e,Optparam)
kp = double(Optparam(1));kd =  double(Optparam(2));ki = double(Optparam(3));b =  double(Optparam(4));m1 =  double(Optparam(5));m2 =  double(Optparam(6));delta =  double(Optparam(7));

%kp = 40;
% kd = 0.2;
% ki = 40;
% alpha = 0.9;
% b = 5.;
% m1 = 10.;
% m2 = 20.;
% delta = 1.;

sdot = -b*s + kp*e + ki*int_e + kd*de;

== matlab function pemfc_lumpekf2_prerun_2/Sliding mode Controller/Controller ==
  data: e input; x input; Grad_fx input; Grad_gx input; fx input; gx input; xdot input; u_eq input; du_eq input; u_S input; du_S input; u_eq_ddot output; sdot input; r input; dr input; ddr input; u_S_ddot output
function [u_eq_ddot,u_S_ddot] = controller(e,x,Grad_fx,Grad_gx,fx,gx,xdot,u_eq,du_eq,u_S,du_S,sdot,r,dr,ddr)
u_eq_ddot = 0;
u_S_ddot = 0;
%% Setting up Control parameter 
kp = 40;
kd = 0.002;
ki = 0.1;
q = 5;
p = 3;
alpha = 0.9;
b = 5.;
m1 = 10.;
m2 = 20.;
delta = 1.;


u = u_eq + u_S;

%% Setting up System parameter 
param.xO2normal = 0.22;
param.BV_Vact0 = 0.0178;
param.J_lim = 30000;
param.BV_J0 = 0.006;
param.Bconc = 0.05;
param.E0_cell = 1.2271;
param.w = 0.05;
param.kE=1.7708e-05;
param.Tfc = 273+33;
	param.r1 = 0.006;
	param.r2 = 4.0000e-05;
	param.rt = 5.0000e-05;
    xch_O2c=0.21;
    param.lc = 1;
    xch_H2a=0.99;
    Pa = 1.5;	%In atm
	Pc = 1; %atm.
J_in = u;
L_zFD=param.xO2normal/param.J_lim;
phi_avg = Pc*xch_O2c;
phiH2_in = Pa*xch_H2a;
phi_eff = 0.1512*phi_avg + 4/pi*x(1) - 4/(3*pi)*x(2) ...
        - (0.1894*J_in + 8/pi^2*x(3))*L_zFD;
J_act = x(5);

temp = [(4/pi)^2,-(1/3)*(4/pi)^2,(4/pi)*(8/pi^2),0,(4/pi)*(-0.1894);
    (1/3)*(4/pi)^2,-(1/9)*(4/pi)^2,(4/pi)*(8/pi^2),0,(4/(3.*pi))*(-0.1894);
    -L_zFD*(4/(pi))*(8/pi^2),-L_zFD*(4/(3.*pi))*(8/pi^2),-L_zFD*(8/(pi))*(8/pi^2),0,-L_zFD*(-0.1894)*(8/pi^2);
    0,0,0,0,0;
     -L_zFD*(-0.1894)*(4/(pi)),-L_zFD*(-0.1894)*(4/(3*pi)),-L_zFD*(-0.1894)*(8/(pi)^2),0,-L_zFD*(-0.1894)*(8/(pi)^2)+2*param.BV_Vact0*J_act/sqrt( 4*param.BV_J0^2 + J_act^2 )];
Gradhxx = u*(-param.Bconc/phi_eff)*temp;
Gradhx = u*[(param.Bconc*(4/pi)/phi_eff);
    (-param.Bconc*(4/(3*pi))/phi_eff);
    (-param.Bconc*(8/pi^2)*L_zFD/phi_eff);
    0;
    -param.Bconc*L_zFD*(0.1894)/(phi_eff) - 2*param.BV_Vact0/sqrt( 4*param.BV_J0^2 + J_act^2 )];
Gradhux = [(param.Bconc*(4/pi)/phi_eff);
    (-param.Bconc*(4/(3*pi))/phi_eff);
    (-param.Bconc*(8/pi^2)*L_zFD/phi_eff);
    0;
    -param.Bconc*L_zFD*(0.1894)/(phi_eff) - 2*param.BV_Vact0/sqrt( 4*param.BV_J0^2 + J_act^2 )];

Area = param.lc*param.w;
I = J_in*Area;
    E0T = param.E0_cell - param.kE*(param.Tfc-298);
    Vact = 2*param.BV_Vact0*asinh(J_act/(2*param.BV_J0));
    if phi_eff<0
        Econc = 0;
    else
        Econc = 2*param.Bconc*log(phiH2_in) + param.Bconc*log(real(phi_eff));
    end
    
    Ecellc =  E0T +  Econc;
    Vohm = (param.r1*I+ param.r2*I^2 - param.rt*(param.Tfc-298)*I); 
    

Gradhu = (Ecellc - Vohm - Vact)+ Area*(param.r1*2.*u+ 3.*param.r2*u^2 - 2.*param.rt*(param.Tfc-298)*u);  
Gradhuu =  Area*(param.r1*2.*u+ 3.*param.r2*u^2 - 2.*param.rt*(param.Tfc-298)*u) + Area*(param.r1*2+ 6*param.r2*u - 2.*param.rt*(param.Tfc-298)); 
Gradhxu = [(param.Bconc*(4/pi)/phi_eff);
    (-param.Bconc*(4/(3*pi))/phi_eff);
    (-param.Bconc*(8/pi^2)*L_zFD/phi_eff);
    0;
    -param.Bconc*L_zFD*(0.1894)/(phi_eff) - 2*param.BV_Vact0/sqrt( 4*param.BV_J0^2 + J_act^2 )];
% t1 = (fx + gx*u_eq)'*Gradhxx*(fx + gx*u_eq)
% t2 = Gradhxx
% t3 = (fx + gx*u_eq)
% t4 = kd*(2*du_eq*Gradhux'*(fx + gx*u_eq) + Gradhx'*(Grad_fx'*xdot + Grad_gx'*xdot*u_eq)+ Gradhuu*du_eq^2-ddr-b*sdot )
% t5 = Gradhx'*(Grad_fx'*xdot + Grad_gx'*xdot*u_eq)
% t6 = Gradhuu*du_eq^2-ddr-b*sdot
% t7 = kp*(Gradhx'*(fx + gx*u_eq)+Gradhu*du_eq - dr)
% t8 = +ki*(sign(e)*abs(e)^(q/p))

u_eq_ddot = -(Gradhu/((Gradhu)^2 + 0.0001))*(kp*(Gradhx'*(fx + gx*u_eq)+Gradhu*du_eq - dr)+ki*(sign(e)*abs(e)^(q/p))+kd*( (fx + gx*u_eq)'*Gradhxx*(fx + gx*u_eq)+...
   2*du_eq*Gradhux'*(fx + gx*u_eq) + Gradhx'*(Grad_fx'*xdot + Grad_gx'*xdot*u_eq)+ Gradhuu*du_eq^2-ddr-b*sdot ));


%%(fx + gx*u_eq)'*Gradhxx*(fx + gx*u_eq)+
%u_eq_ddot = -(Gradhu/((Gradhu)^2 + 0.0001))*(kp*(Gradhx'*(fx + gx*u_eq)+Gradhu*du_eq - dr)+ki*(sign(e)*abs(e)^(q/p))+kd*((fx + gx*u_eq)'*Gradhxx*(fx + gx*u_eq)+ ...
%    2*du_eq*Gradhux'*(fx + gx*u_eq) + Gradhx'*(Grad_fx'*xdot + Grad_gx'*xdot*u_eq)+ Gradhuu*du_eq^2-ddr-b*sdot ))
%u_eq_ddot = 0;
u_S_ddot =  -(Gradhu/((Gradhu)^2 + 0.0001))*(kp*(Gradhx'*(gx*u_S)+Gradhu*du_S)+kd*((gx*u_S)'*Gradhxx*(gx*u_S))+(gx*u_S)'*Gradhxu*du_S ...
    +Gradhuu*du_S^2+Gradhx'*(Grad_gx'*xdot)*u_S+m1*abs(sdot)*sign(sdot)+m2*sign(sdot)*abs(sdot)^alpha+delta*sign(sdot));
